simulink model "sharedControlWRos"  (R2018a)
settings: Solver=VariableStepAuto  StartTime=0.0  StopTime=200  RelTol=1e-3
InitFcn:
  | load('joystick_ref_002.mat')
  | % global t_change;
  | % t_change=0;
  | 
  | % T = 20;
  | a = 0.5;
  | b = 1;
  | v0 = 1;
  | tau = 0.5;
  | %tau=10;
  | 
  | % PID Gains
  | % kp = 10;
  | kp = 2*b/a^2;
  | TI = 5;
  | TD = 0.1;
  | 
  | % SM Gains
  | k0 = 20;
  | k1 = 0.05;
  | 
  | % DAS
  | DT=4;
  | % gamma1sq=0.05;
  | % gamma2sq=0.3;
  | gamma1sq=0.2;
  | gamma2sq=0.1;
  | y_ref=0;
  | 
  | initSub = rossubscriber('/ship/state');
  | initMsg = receive(initSub,10)
  | 
  | Yd_init=initMsg.Pose.X
values from neighbouring files (symbols this model uses):
  a2 = 26.4940946148    [CrossTrackUSV.mat]
  b2 = 0.266666666667    [CrossTrackUSV.mat]
  K2 = 1219.40576956    [CrossTrackUSV.mat]
libraries: robotlib x3, vrlib x1, realtime_pacer_lib x1
settings Model: Creator=transmogrifier  LastModifiedBy=transmogrifier

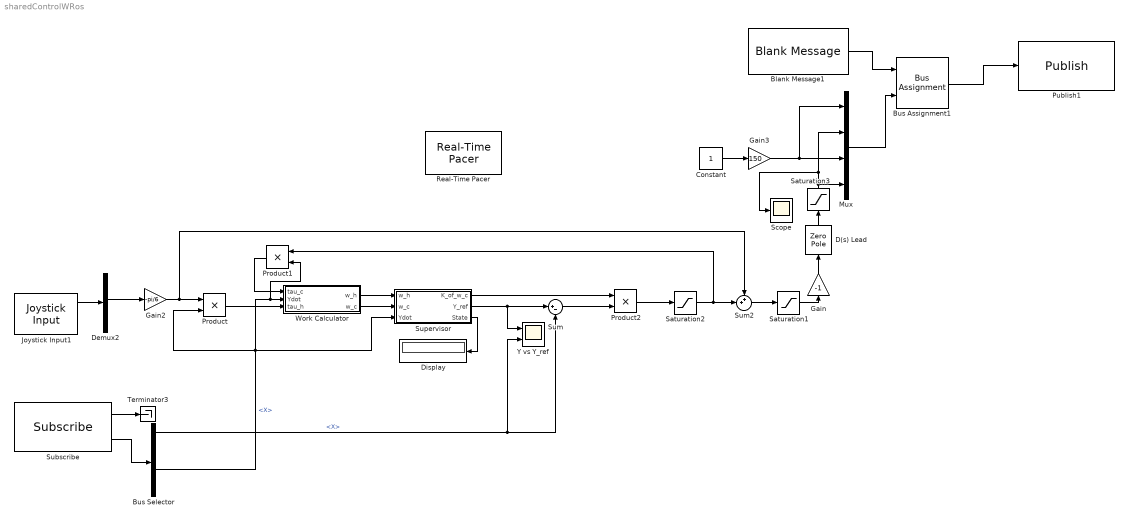
== system sharedControlWRos ==
  Blank Message1 : robotlib/Blank Message  SourceLibraryInfo=This block requires Robotics System Toolbox  messageType=usv16_msgs/Usv16ActuatorInputs  SampleTime=inf
      settings: SourceProductBaseCode=RO
  Bus Assignment1 : BusAssignment  AssignedSignals=ActuatorInputs
  Bus Selector : BusSelector  OutputSignals=Pose.X,Pose.Y,Vel.Linear.X,Vel.Linear.Y
  Constant : Constant
  D(s) Lead : ZeroPole  Zeros=[-b2]  Poles=[-a2]  Gain=[K2]
  Demux2 : Demux  Outputs=8
  Display : Display
  Gain : Gain  Gain=-1
  Gain2 : Gain  Gain=-pi/6
  Gain3 : Gain  Gain=150
  Joystick Input1 : vrlib/Joystick Input  joyid=1  adjustports=on  forcefeed=off
      settings: SourceProductBaseCode=VR
  Mux : Mux
  Product : Product
  Product1 : Product
  Product2 : Product
  Publish1 : robotlib/Publish  SourceLibraryInfo=This block requires Robotics System Toolbox  topicSource=Select from ROS network  topic=/ship/actuation  messageType=usv16_msgs/Usv16ActuatorInputs  messageQueueLength=1
      settings: SourceProductBaseCode=RO
  Real-Time Pacer : realtime_pacer_lib/Real-Time Pacer  simTimePerRealTime=1
  Saturation1 : Saturate  UpperLimit=pi/6  LowerLimit=-pi/6
  Saturation2 : Saturate  UpperLimit=pi/6  LowerLimit=-pi/6
  Saturation3 : Saturate  UpperLimit=pi/6  LowerLimit=-pi/6
  Scope : Scope
  Subscribe : robotlib/Subscribe  SourceLibraryInfo=This block requires Robotics System Toolbox  topicSource=Select from ROS network  topic=/ship/state  messageType=usv16_msgs/Usv16State  sampleTime=-1  messageQueueLength=1
      settings: SourceProductBaseCode=RO
  Sum : Sum  Inputs=|+-
  Sum2 : Sum  Inputs=++|
  Supervisor : Subsystem  mask{gamma_1_sq=0.2, gamma_2_sq=0.1, a_d=10, b_d=0.4, sigma_sq=0.1, delta_y=4, K3=0.5}
      mask prompts: gamma_1_sq "DAS Threshold"; gamma_2_sq "Human Threshold"; a_d "a"; b_d "b"; sigma_sq "Lane Change Threshold"; delta_y "Lane Change Delta"; K3 "K0"
  Terminator3 : Terminator
  Work Calculator : Subsystem  mask{DT=4}
      mask prompts: DT "Time Window"
  Y vs Y_ref : Scope  NumInputPorts=2
  wires:
  Subscribe/1 -> Terminator3/1
  Supervisor/2(Y_ref) -> Y vs Y_ref/1, Sum/1
  Saturation2/1 -> Sum2/2, Product1/1
  Sum2/1 -> Saturation1/1
  Gain3/1 -> Mux/1, Mux/3
  Product2/1 -> Saturation2/1
  Bus Assignment1/1 -> Publish1/1
  Mux/1 -> Bus Assignment1/2
  Saturation1/1 -> Gain/1
  Bus Selector/1 -> Y vs Y_ref/2, Sum/2  "<X>"
  Bus Selector/3 -> Supervisor/3(Ydot), Product1/2, Work Calculator/2(Ydot), Product/2  "<X>"
  Subscribe/2 -> Bus Selector/1
  Work Calculator/1(w_h) -> Supervisor/1(w_h)
  Work Calculator/2(w_c) -> Supervisor/2(w_c)
  Gain2/1 -> Sum2/1, Product/1
  Constant/1 -> Gain3/1
  Supervisor/3(State) -> Display/1
  Blank Message1/1 -> Bus Assignment1/1
  Joystick Input1/1 -> Demux2/1
  Product/1 -> Work Calculator/3(tau_h)
  Product1/1 -> Work Calculator/1(tau_c)
  Sum/1 -> Product2/2
  Demux2/4 -> Gain2/1
  Supervisor/1(K_of_w_c) -> Product2/1
  D(s) Lead/1 -> Saturation3/1
  Gain/1 -> D(s) Lead/1
  Saturation3/1 -> Scope/1, Mux/2, Mux/4

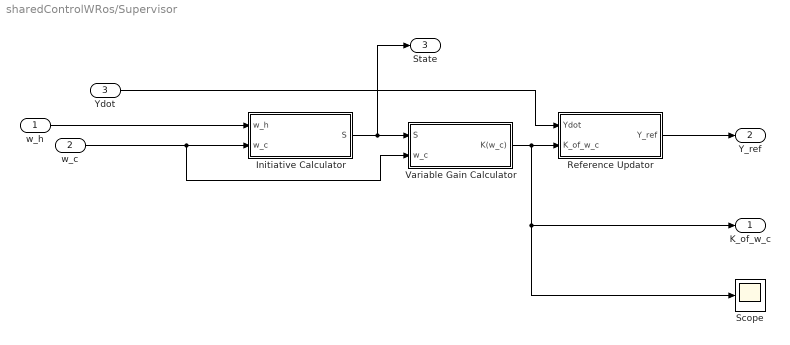
== system sharedControlWRos/Supervisor ==
  w_h : Inport
  w_c : Inport  Port=2
  Ydot : Inport  Port=3
  Initiative Calculator : Subsystem
  Reference Updator : Subsystem
  Scope : Scope
  Variable Gain Calculator : Subsystem
  K_of_w_c : Outport
  Y_ref : Outport  Port=2
  State : Outport  Port=3
  wires:
  w_c/1 -> Variable Gain Calculator/2(w_c), Initiative Calculator/2("w_c ")
  w_h/1 -> Initiative Calculator/1(w_h)
  Initiative Calculator/1(S) -> State/1, Variable Gain Calculator/1(S)
  Variable Gain Calculator/1(K(w_c)) -> Reference Updator/2(K_of_w_c), Scope/1, K_of_w_c/1
  Ydot/1 -> Reference Updator/1(Ydot)
  Reference Updator/1(Y_ref) -> Y_ref/1

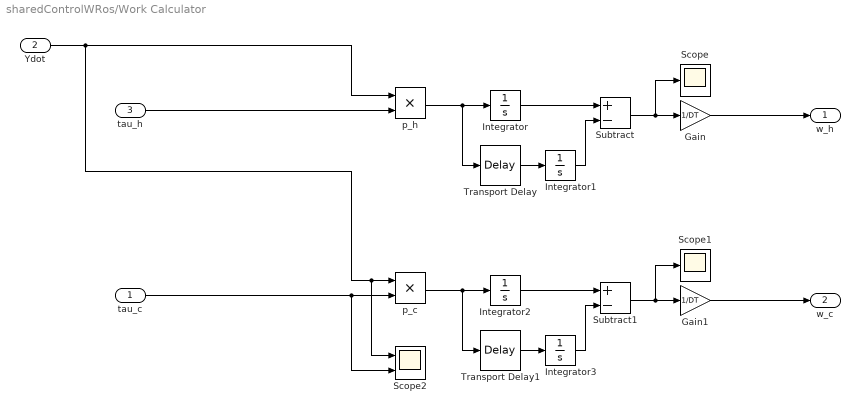
== system sharedControlWRos/Work Calculator ==
  tau_c : Inport
  Ydot : Inport  Port=2
  tau_h : Inport  Port=3
  Gain : Gain  Gain=1/DT
  Gain1 : Gain  Gain=1/DT
  Integrator{,1..3} (4 alike) : Integrator
  Scope : Scope
  Scope1 : Scope
  Scope2 : Scope  NumInputPorts=2
  Subtract : Sum  Inputs=+-
  Subtract1 : Sum  Inputs=+-
  Transport Delay : TransportDelay  DelayTime=DT
  Transport Delay1 : TransportDelay  DelayTime=DT
  p_c : Product
  p_h : Product
  w_h : Outport
  w_c : Outport  Port=2
  wires:
  tau_c/1 -> Scope2/2, p_c/2
  tau_h/1 -> p_h/2
  p_h/1 -> Transport Delay/1, Integrator/1
  Subtract/1 -> Scope/1, Gain/1
  Ydot/1 -> p_h/1, Scope2/1, p_c/1
  Transport Delay/1 -> Integrator1/1
  Integrator/1 -> Subtract/1
  Integrator1/1 -> Subtract/2
  Gain/1 -> w_h/1
  p_c/1 -> Transport Delay1/1, Integrator2/1
  Transport Delay1/1 -> Integrator3/1
  Subtract1/1 -> Scope1/1, Gain1/1
  Integrator2/1 -> Subtract1/1
  Integrator3/1 -> Subtract1/2
  Gain1/1 -> w_c/1

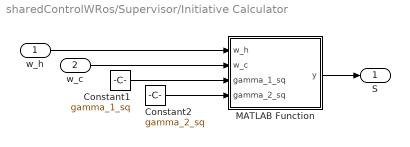
== system sharedControlWRos/Supervisor/Initiative Calculator ==
  w_h : Inport
  "w_c " : Inport  Port=2
  Constant1 : Constant  Value=gamma_1_sq
  Constant2 : Constant  Value=gamma_2_sq
  MATLAB Function : MATLAB Function  TreatAsAtomicUnit=on
  S : Outport
  wires:
  w_h/1 -> MATLAB Function/1(w_h)
  MATLAB Function/1(y) -> S/1
  Constant2/1 -> MATLAB Function/4(gamma_2_sq)
  "w_c "/1 -> MATLAB Function/2(w_c)
  Constant1/1 -> MATLAB Function/3(gamma_1_sq)

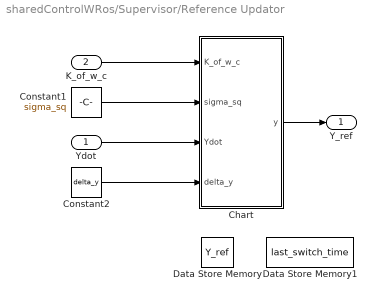
== system sharedControlWRos/Supervisor/Reference Updator ==
  Ydot : Inport
  K_of_w_c : Inport  Port=2
  Chart : Stateflow chart  TreatAsAtomicUnit=on
  Constant1 : Constant  Value=sigma_sq
  Constant2 : Constant  Value=delta_y
  Data Store Memory : DataStoreMemory  DataStoreName=Y_ref  ReadBeforeWriteMsg=warning  WriteAfterWriteMsg=warning  WriteAfterReadMsg=warning  ShowAdditionalParam=off  OutDataTypeStr=int16
  Data Store Memory1 : DataStoreMemory  DataStoreName=last_switch_time  ReadBeforeWriteMsg=warning  WriteAfterWriteMsg=warning  WriteAfterReadMsg=warning  ShowAdditionalParam=off  OutDataTypeStr=double
  Y_ref : Outport
  wires:
  Ydot/1 -> Chart/3(Ydot)
  K_of_w_c/1 -> Chart/1(K_of_w_c)
  Chart/1(y) -> Y_ref/1
  Constant1/1 -> Chart/2(sigma_sq)
  Constant2/1 -> Chart/4(delta_y)

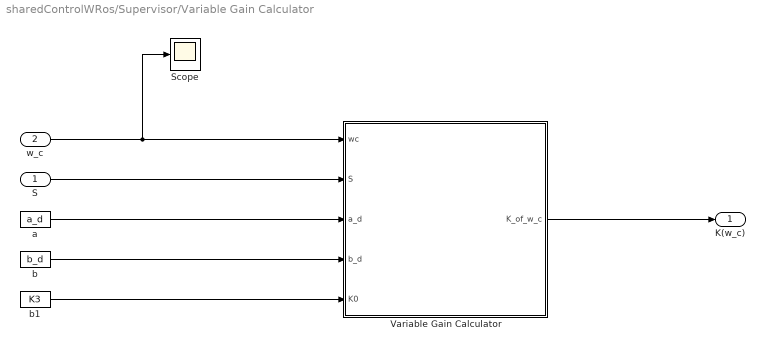
== system sharedControlWRos/Supervisor/Variable Gain Calculator ==
  S : Inport
  w_c : Inport  Port=2
  Scope : Scope
  "Variable Gain Calculator " : MATLAB Function  TreatAsAtomicUnit=on
  a : Constant  Value=a_d
  b : Constant  Value=b_d
  b1 : Constant  Value=K3
  K(w_c) : Outport
  wires:
  "Variable Gain Calculator "/1(K_of_w_c) -> K(w_c)/1
  a/1 -> "Variable Gain Calculator "/3(a_d)
  w_c/1 -> Scope/1, "Variable Gain Calculator "/1(wc)
  S/1 -> "Variable Gain Calculator "/2(S)
  b/1 -> "Variable Gain Calculator "/4(b_d)
  b1/1 -> "Variable Gain Calculator "/5(K0)

== stateflow chart sharedControlWRos/Supervisor/Reference Updator/Chart ==
  note: This system will check if there should be a lane changed
      | based on K(w_c) vs siqma^2.  If a lane change is required,
      | check to see if allowed based on time since last lane change
  note: C style logic:
      | if(K_of_w_c<=sigma_sq)
      | if(Ydot>0)
      | Y_ref=Y_ref+delta_y;
      | elseif(Ydot<0)
      | Y_ref=Y_ref-delta_y;
      | end
      | end
      | y = Y_ref;
  state add
    entry:Y_ref=Y_ref+delta_y;
    y=Y_ref;
    set_last_switch_time;
  state checkForChange
    entry: change_flag=time_check(20);
  state subtract
    entry:Y_ref=Y_ref-delta_y;
    y=Y_ref;
    set_last_switch_time;
  note: T_min=5
  add -> checkForChange
  (default) -> checkForChange
  (junction 47) -> add [order 1] : [Ydot>0]
  checkForChange -> (junction 44) [order 1] : [change_flag==true]
  (junction 44) -> (junction 47) [order 1] : [(K_of_w_c<=sigma_sq)]
  (junction 44) -> checkForChange [order 2] : [(K_of_w_c>sigma_sq)]
  (junction 47) -> subtract [order 2] : [Ydot<0]
  checkForChange -> checkForChange [order 2] : [change_flag==false]
  subtract -> checkForChange
  data: change function_output; t_min function_input; K_of_w_c input; sigma_sq input; y output; Ydot input; delta_y input; Y_ref data_store_memory; last_switch_time data_store_memory; current_time local; change_flag local
  function change=time_check(t_min):
    | function change=time_check(t_min)
    | global last_switch_time
    | coder.extrinsic('get_param');
    | temp=0;
    | temp=get_param('sharedControlWRos','SimulationTime');
    | change=(temp-last_switch_time)>t_min;
  function set_last_switch_time:
    | function set_last_switch_time
    | global last_switch_time
    | coder.extrinsic('get_param')
    | last_switch_time=get_param('sharedControlWRos','SimulationTime');

== matlab function sharedControlWRos/Supervisor/Initiative Calculator/MATLAB Function ==
  data: w_h input; y output; w_c input; gamma_1_sq input; gamma_2_sq input
function y = fcn(w_h, w_c, gamma_1_sq, gamma_2_sq)

if(w_h >= -gamma_1_sq && w_c >= -gamma_2_sq)
    S=1;
elseif(w_h >= -gamma_1_sq && w_c < -gamma_2_sq)
    S=2;
elseif(w_h < -gamma_1_sq && w_c >= -gamma_2_sq)
    S=3;
elseif(w_h < -gamma_1_sq && w_c < -gamma_2_sq)
    S=4;
else
    error('bad state assignment');
end
y = S;

== matlab function sharedControlWRos/Supervisor/Variable Gain Calculator/Variable Gain Calculator  ==
  data: wc input; S input; K_of_w_c output; a_d input; b_d input; K0 input
function K_of_w_c = fcn(wc, S, a_d, b_d, K0)

if S == 2    
    K_of_w_c = K0/(1 + exp(-a_d*wc + b_d));
else
    K_of_w_c = K0;
end

return
